simulink model "F_task"  (R2024a)
settings: Solver=VariableStepAuto  StartTime=0.0  StopTime=5  RelTol=1e-3
PreLoadFcn:
  | fs=3.2e6;
StartFcn:
  | fs=3.2e6;
undefined symbols (not defined in the file): designMultirateFIR
libraries: dspmlti4 x2, rtlsdr_book_library x2
settings Model: Creator=wluha  LastModifiedBy=april
settings RTWCC: GPUComputeCapability=3.5

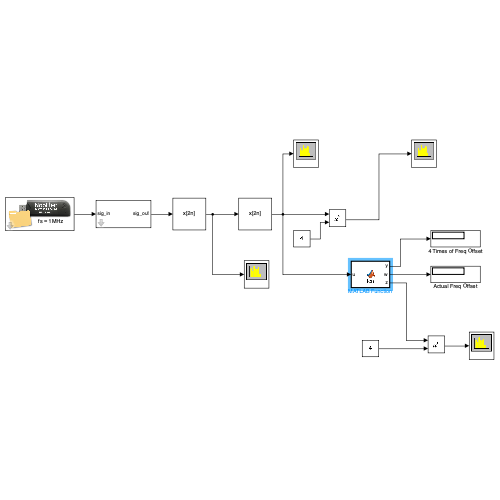
[thumbnail: Simulink's stored preview of the top-level diagram]
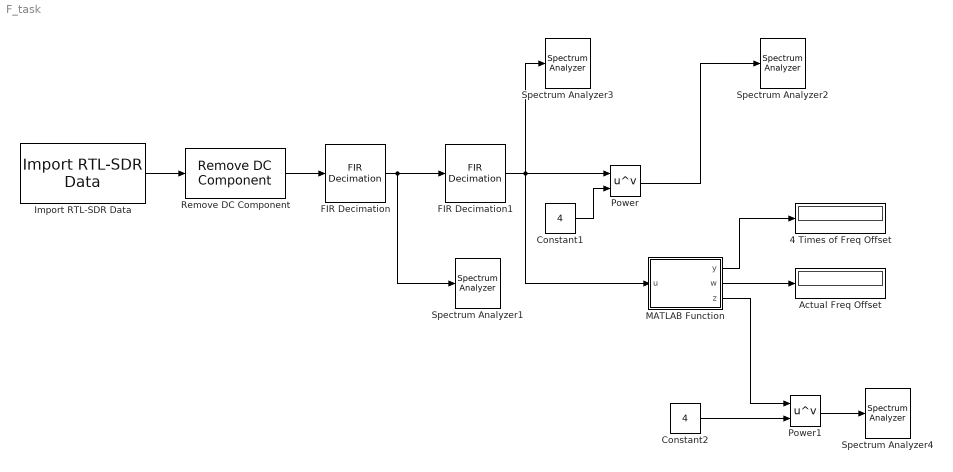
== system F_task ==
  4 Times of Freq Offset : Display
  Actual Freq Offset : Display
  Constant1 : Constant  Value=4
  Constant2 : Constant  Value=4
  FIR Decimation : dspmlti4/FIR Decimation  FilterSource=Auto  h=designMultirateFIR(1,2)  D=2  filtStruct=Direct form  FilterObject=FDECIM  InputProcessing=Columns as channels (frame based)  framing=Enforce single-rate processing  AllowArbitraryInputLength=off  inputOffset=0  outputBufInitCond=0  roundingMode=Floor  overflowMode=off  firstCoeffDataTypeStr=Inherit: Same word length as input  firstCoeffMin=[]  firstCoeffMax=[]  firstCoeffLastDataTypeStr=Inherit: Same word length as input  outputDataTypeStr=Inherit: Same as accumulator  outputMin=[]  outputMax=[]  outputLastDataTypeStr=Inherit: Same as accumulator
  FIR Decimation1 : dspmlti4/FIR Decimation  FilterSource=Auto  h=designMultirateFIR(1,2)  D=2  filtStruct=Direct form  FilterObject=FDECIM  InputProcessing=Columns as channels (frame based)  framing=Enforce single-rate processing  AllowArbitraryInputLength=off  inputOffset=0  outputBufInitCond=0  roundingMode=Floor  overflowMode=off  firstCoeffDataTypeStr=Inherit: Same word length as input  firstCoeffMin=[]  firstCoeffMax=[]  firstCoeffLastDataTypeStr=Inherit: Same word length as input  outputDataTypeStr=Inherit: Same as accumulator  outputMin=[]  outputMax=[]  outputLastDataTypeStr=Inherit: Same as accumulator
  Import RTL-SDR Data : rtlsdr_book_library/Additional Tools/Import RTL-SDR Data  filename=/Users/april/Desktop/2026下半学期作业/通信建模与仿真/粗频偏估计和测量/rtlsdr_data_435MHz_1MHz_Sampling_01.mat  frm_size=4096  data_type=double
      settings: SourceProductName=RTL-SDR Book Library
  MATLAB Function : MATLAB Function  TreatAsAtomicUnit=on
  Power : Math  Operator=pow
  Power1 : Math  Operator=pow
  Remove DC Component : rtlsdr_book_library/Additional Tools/Remove DC Component
      settings: SourceProductName=RTL-SDR Book Library
  Spectrum Analyzer1 : SpectrumAnalyzer  WindowPosition=[79.000000,31.000000,819.000000,475.000000,]  Visible=on  ScopeFrameLocation=window  Span=2000000.0000000002  StartFrequency=-1000000.0000000001  StopFrequency=1000000.0000000001  YLimits=[-44.30247353,21.77394197]  SelectedToolstripTab=spectrumAnalyzerToolstrip.measurementsTab
  Spectrum Analyzer2 : SpectrumAnalyzer  WindowPosition=[8.000000,80.000000,1426.000000,792.000000,]  Visible=on  ScopeFrameLocation=window  Span=2000000.0000000002  StartFrequency=-1000000.0000000001  StopFrequency=1000000.0000000001  YLimits=[-39.52239608,28.14030333]  SelectedToolstripTab=spectrumAnalyzerToolstrip.measurementsTab
  Spectrum Analyzer3 : SpectrumAnalyzer  WindowPosition=[8.000000,80.000000,1426.000000,792.000000,]  Visible=on  ScopeFrameLocation=window  Span=2000000.0000000002  StartFrequency=-1000000.0000000001  StopFrequency=1000000.0000000001  YLimits=[-47.99653355,22.21018503]  SelectedToolstripTab=spectrumAnalyzerToolstrip.measurementsTab
  Spectrum Analyzer4 : SpectrumAnalyzer  WindowPosition=[1.000000,91.000000,1440.000000,805.000000,]  Visible=on  ScopeFrameLocation=window  Span=2000000.0000000002  StartFrequency=-1000000.0000000001  StopFrequency=1000000.0000000001  YLimits=[-39.51901062557098,27.865620616683792]  SelectedToolstripTab=spectrumAnalyzerToolstrip.measurementsTab
  wires:
  FIR Decimation/1 -> Spectrum Analyzer1/1, FIR Decimation1/1
  FIR Decimation1/1 -> MATLAB Function/1(u), Power/1, Spectrum Analyzer3/1
  Constant1/1 -> Power/2
  Power/1 -> Spectrum Analyzer2/1
  MATLAB Function/1(y) -> 4 Times of Freq Offset/1
  MATLAB Function/3(z) -> Power1/1
  Constant2/1 -> Power1/2
  Power1/1 -> Spectrum Analyzer4/1
  MATLAB Function/2(w) -> Actual Freq Offset/1
  Import RTL-SDR Data/1 -> Remove DC Component/1
  Remove DC Component/1 -> FIR Decimation/1

== matlab function F_task/MATLAB Function ==
  data: u input; y output; w output; z output
function [y,w,z]= fcn(u)
quard_u = u.^4;
Nfft = 2048;
fs_1 = 1e6/4;
[v, i] = max(abs(fftshift(fft(quard_u, Nfft))));
spectrum_peak =  i- Nfft/2; 

foffset = fs_1 / Nfft * spectrum_peak;

y = foffset;
w = foffset / 4;
u_move = circshift(fft(u,Nfft),-1* round(spectrum_peak/4));
z = ifft(u_move);
